simulink model "Kalman_Phase_Simple"  (R2019b)
settings: Solver=VariableStepAuto  StartTime=0.0  StopTime=model.sim_dur  FixedStep=model.Ts  RelTol=1e-6
values from neighbouring files (symbols this model uses):
  D = 0    [Kalman.m]
undefined symbols (not defined in the file or in its folder): model
libraries: dspsrcs4 x5, dspindex x2
settings Model: Creator=isidoraradenkovic  LastModifiedBy=isidoraradenkovic

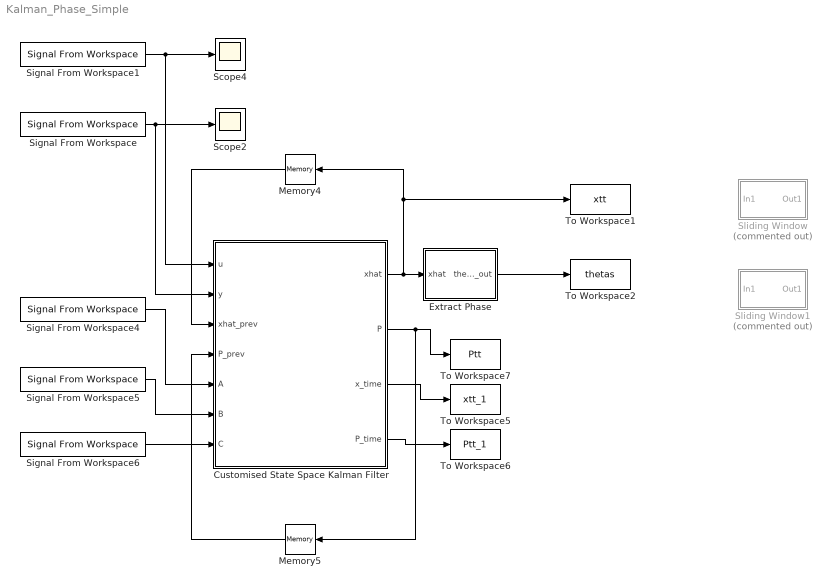
== system Kalman_Phase_Simple ==
  Customised State Space Kalman Filter : MATLAB Function  TreatAsAtomicUnit=on
  Extract Phase : MATLAB Function  TreatAsAtomicUnit=on  SystemSampleTime=model.Ts
  Memory4 : Memory  InitialCondition=model.x_0  InheritSampleTime=on
  Memory5 : Memory  InitialCondition=model.Q  InheritSampleTime=on
  Scope2 : Scope
  Scope4 : Scope
  Signal From Workspace : dspsrcs4/Signal From Workspace  X=input_data  Ts=model.Ts  nsamps=1  OutputAfterFinalValue=Cyclic repetition  ignoreOrWarnInputAndFrameLengths=off  OutputFrames=off
  Signal From Workspace1 : dspsrcs4/Signal From Workspace  X=tms_pulses  Ts=model.Ts  nsamps=1  OutputAfterFinalValue=Cyclic repetition  ignoreOrWarnInputAndFrameLengths=off  OutputFrames=off
  Signal From Workspace4 : dspsrcs4/Signal From Workspace  X=model.A  Ts=model.Ts/2  nsamps=2  OutputAfterFinalValue=Cyclic repetition  ignoreOrWarnInputAndFrameLengths=off  OutputFrames=off
  Signal From Workspace5 : dspsrcs4/Signal From Workspace  X=model.B  Ts=model.Ts/2  nsamps=2  OutputAfterFinalValue=Cyclic repetition  ignoreOrWarnInputAndFrameLengths=off  OutputFrames=off
  Signal From Workspace6 : dspsrcs4/Signal From Workspace  X=model.C  Ts=model.Ts  nsamps=1  OutputAfterFinalValue=Cyclic repetition  ignoreOrWarnInputAndFrameLengths=off  OutputFrames=off
  Sliding Window : Subsystem  Commented=on
  Sliding Window1 : Subsystem  Commented=on
  To Workspace1 : ToWorkspace  VariableName=xtt  SampleTime=model.Ts
      settings: Save2DSignal=2-D array (concatenate along first dimension)
  To Workspace2 : ToWorkspace  VariableName=thetas  SampleTime=model.Ts
      settings: Save2DSignal=2-D array (concatenate along first dimension)
  To Workspace5 : ToWorkspace  VariableName=xtt_1  SampleTime=model.Ts
      settings: Save2DSignal=2-D array (concatenate along first dimension)
  To Workspace6 : ToWorkspace  VariableName=Ptt_1  SampleTime=model.Ts
      settings: Save2DSignal=2-D array (concatenate along first dimension)
  To Workspace7 : ToWorkspace  VariableName=Ptt  SampleTime=model.Ts
      settings: Save2DSignal=2-D array (concatenate along first dimension)
  wires:
  Customised State Space Kalman Filter/2(P) -> To Workspace7/1, Memory5/1
  Customised State Space Kalman Filter/4(P_time) -> To Workspace6/1
  Signal From Workspace6/1 -> Customised State Space Kalman Filter/7(C)
  Signal From Workspace5/1 -> Customised State Space Kalman Filter/6(B)
  Signal From Workspace/1 -> Customised State Space Kalman Filter/2(y), Scope2/1
  Customised State Space Kalman Filter/3(x_time) -> To Workspace5/1
  Signal From Workspace4/1 -> Customised State Space Kalman Filter/5(A)
  Signal From Workspace1/1 -> Customised State Space Kalman Filter/1(u), Scope4/1
  Customised State Space Kalman Filter/1(xhat) -> To Workspace1/1, Memory4/1, Extract Phase/1(xhat)
  Memory5/1 -> Customised State Space Kalman Filter/4(P_prev)
  Memory4/1 -> Customised State Space Kalman Filter/3(xhat_prev)
  Extract Phase/1(thetas_out) -> To Workspace2/1

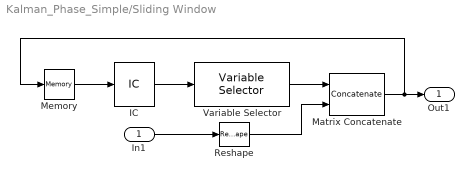
== system Kalman_Phase_Simple/Sliding Window ==
  In1 : Inport
  IC : InitialCondition  Value=zeros(model.window, 2)
  Matrix Concatenate : Concatenate  Mode=Multidimensional array
  Memory : Memory  InheritSampleTime=on
  Reshape : Reshape  OutputDimensionality=Row vector (2-D)
  Variable Selector : dspindex/Variable Selector  NumInputs=1  rowsOrCols=Rows  IdxMode=Fixed  Elements=2:model.window  ZerOneIdxMode=One-based  errmode=Clip Index  FillMode=on  FillValues=0
  Out1 : Outport
  wires:
  Matrix Concatenate/1 -> Memory/1, Out1/1
  IC/1 -> Variable Selector/1
  Memory/1 -> IC/1
  In1/1 -> Reshape/1
  Variable Selector/1 -> Matrix Concatenate/1
  Reshape/1 -> Matrix Concatenate/2

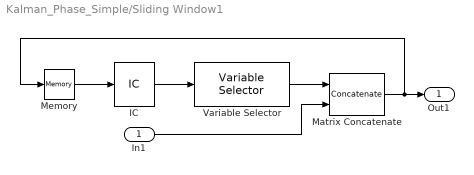
== system Kalman_Phase_Simple/Sliding Window1 ==
  In1 : Inport
  IC : InitialCondition  Value=zeros(model.window, 1)
  Matrix Concatenate : Concatenate  Mode=Multidimensional array
  Memory : Memory  InheritSampleTime=on
  Variable Selector : dspindex/Variable Selector  NumInputs=1  rowsOrCols=Rows  IdxMode=Fixed  Elements=2:model.window  ZerOneIdxMode=One-based  errmode=Clip Index  FillMode=on  FillValues=0
  Out1 : Outport
  wires:
  Matrix Concatenate/1 -> Memory/1, Out1/1
  IC/1 -> Variable Selector/1
  Memory/1 -> IC/1
  Variable Selector/1 -> Matrix Concatenate/1
  In1/1 -> Matrix Concatenate/2

== matlab function Kalman_Phase_Simple/Extract Phase ==
  settings: updateMethod=DISCRETE  sampleTime=model.Ts
  data: xhat input; thetas_out output
function thetas_out  = extract_phase(xhat)
num_rhythms = length(xhat)/2;
% thetas_out = zeros(num_rhythms, 1);
% 
% for j = 1:num_rhythms
%     Im = xhat(2 * (j-1) + 2);
%     Re = xhat(2 * (j-1) + 1);
%     thetas_out(j, 1) = atan2(Im, Re);
% end

thetas_out = atan2(xhat(2:2:2*num_rhythms), xhat(1:2:2*(num_rhythms-1)+1))

== matlab function Kalman_Phase_Simple/Customised State Space Kalman Filter ==
  data: u input; xhat output; y input; xhat_prev input; P_prev input; A input; B input; C input; P output; x_time output; P_time output; model parameter
function [xhat, P, x_time, P_time] = custom_state_space_kalman(u, y, xhat_prev, P_prev, A, B, C, model)
x_time = A*xhat_prev + B*u;
P_time = A*P_prev*A'+ model.Gm*model.Q*model.Gm';

K = P_time*(C')*pinv(C*P_time*C' + model.R);
epsilon = y - C*x_time;

xhat = x_time + K*epsilon;
P = P_time - K*C*P_time;
end
